simulink model "model"  (R2022a)
settings: Solver=VariableStepAuto  StartTime=0.0  StopTime=simtime  RelTol=1e-3
model workspace (MAT data in the model file):
  simtime = 3
values from neighbouring files (symbols this model uses):
  AVeh = 1.05    [first_test.mat]    (also in malgucka.m)
  coeffAir = 1.35    [first_test.mat]    (also in malgucka.m)
  coeffGrvy = 9.81    [first_test.mat]    (also in malgucka.m)
  coeffLift = 5.2    [first_test.mat]    (also in malgucka.m)
  coeffRoll = 0.025    [first_test.mat]    (also in malgucka.m)
  densAir = 1.225    [first_test.mat]    (also in malgucka.m)
  dstRdTir = 0.2032    [first_test.mat]    (also in malgucka.m)
  gbx = 16    [first_test.mat]    (also in malgucka.m = 13.11)
  initial_speed = max(v_acc) / 3.6    [laptimeV1.m]
  mTir = 5.3    [first_test.mat]    (also in malgucka.m)
  mVeh = 282    [first_test.mat]    (also in malgucka.m)
  tq_Mot_Re = [40 40 40 40 40 40 40 40 40 40 40 40 ... (46 elements, 1x46)]    [first_test.mat]    (also in laptimeV1.m = [0 0 0 0 0 0 0])
settings Model: Creator=gbour  LastModifiedBy=gbour
settings DebuggingCC: AlgebraicLoopMsg=none

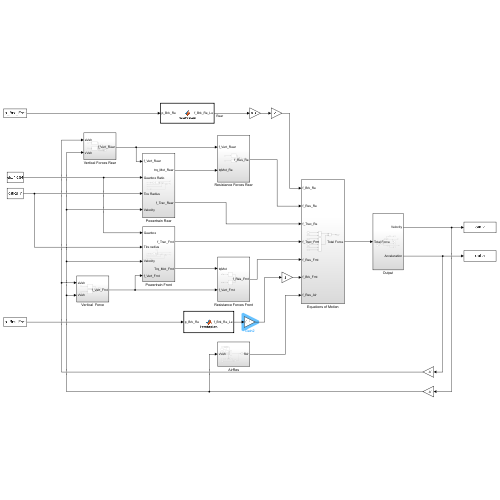
[thumbnail: Simulink's stored preview of the top-level diagram]
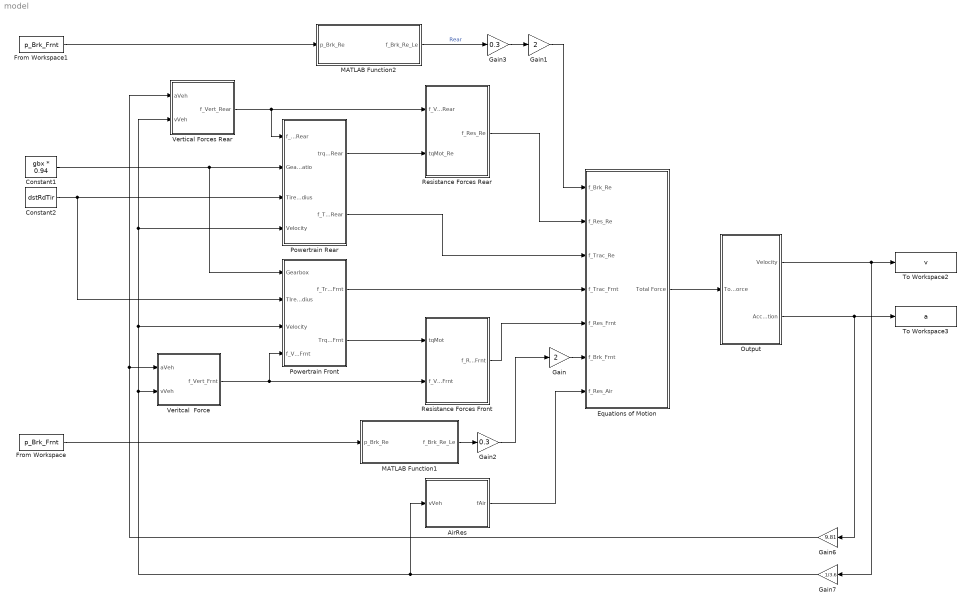
== system model ==
  AirRes : Subsystem
  Constant1 : Constant  Value=gbx * 0.94
  Constant2 : Constant  Value=dstRdTir
  Equations of Motion : Subsystem
  From Workspace : FromWorkspace  VariableName=p_Brk_Frnt
  From Workspace1 : FromWorkspace  VariableName=p_Brk_Frnt
  Gain : Gain  Gain=2
  Gain1 : Gain  Gain=2
  Gain2 : Gain  Gain=0.3
  Gain3 : Gain  Gain=0.3
  Gain6 : Gain  Gain=9.81
  Gain7 : Gain  Gain=1/3.6
  MATLAB Function1 : MATLAB Function  TreatAsAtomicUnit=on
  MATLAB Function2 : MATLAB Function  TreatAsAtomicUnit=on
  Output : Subsystem
  Powertrain Front : Subsystem
  Powertrain Rear : Subsystem
  Resistance Forces Front : Subsystem
  Resistance Forces Rear : Subsystem
  To Workspace2 : ToWorkspace  VariableName=v  SampleTime=-1
      settings: Save2DSignal=2-D array (concatenate along first dimension)
  To Workspace3 : ToWorkspace  VariableName=a  SampleTime=-1
      settings: Save2DSignal=2-D array (concatenate along first dimension)
  Veritcal  Force : Subsystem
  Vertical Forces Rear : Subsystem
  wires:
  Constant1/1 -> Powertrain Front/1(Gearbox), Powertrain Rear/2(Gearbox Ratio)
  Constant2/1 -> Powertrain Rear/3(Tire Radius), Powertrain Front/2(TIre radius)
  Output/1(Velocity) -> To Workspace2/1, Gain7/1
  Output/2(Acceleration) -> To Workspace3/1, Gain6/1
  Equations of Motion/1(Total Force) -> Output/1(Total Force)
  Resistance Forces Front/1(f_Res_Frnt) -> Equations of Motion/5(f_Res_Frnt)
  Veritcal  Force/1(f_Vert_Frnt) -> Powertrain Front/4(f_Vert_Frnt), Resistance Forces Front/2(f_Vert_Frnt)
  Powertrain Front/1(f_Trac_Frnt) -> Equations of Motion/4(f_Trac_Frnt)
  Powertrain Front/2(Trq_Mot_Frnt) -> Resistance Forces Front/1(tqMot)
  AirRes/1(fAir) -> Equations of Motion/7(f_Res_Air)
  Powertrain Rear/2(f_Trac_Rear) -> Equations of Motion/3(f_Trac_Re)
  Vertical Forces Rear/1(f_Vert_Rear) -> Resistance Forces Rear/1(f_Vert_Rear), Powertrain Rear/1(f_Vert_Rear)
  Powertrain Rear/1(trq_Mot_Rear) -> Resistance Forces Rear/2(tqMot_Re)
  Resistance Forces Rear/1(f_Res_Re) -> Equations of Motion/2(f_Res_Re)
  Gain6/1 -> Vertical Forces Rear/1(aVeh), Veritcal  Force/1(aVeh)
  Gain7/1 -> Powertrain Front/3(Velocity), Powertrain Rear/4(Velocity), Vertical Forces Rear/2(vVeh), Veritcal  Force/2(vVeh), AirRes/1(vVeh)
  MATLAB Function1/1(f_Brk_Re_Le) -> Gain2/1
  From Workspace/1 -> MATLAB Function1/1(p_Brk_Re)
  From Workspace1/1 -> MATLAB Function2/1(p_Brk_Re)
  MATLAB Function2/1(f_Brk_Re_Le) -> Gain3/1  "Rear"
  Gain/1 -> Equations of Motion/6(f_Brk_Frnt)
  Gain1/1 -> Equations of Motion/1(f_Brk_Re)
  Gain2/1 -> Gain/1
  Gain3/1 -> Gain1/1

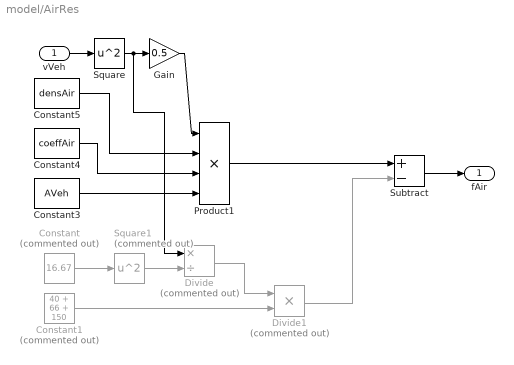
== system model/AirRes ==
  vVeh : Inport
  Constant : Constant  Commented=on  Value=16.67
  Constant1 : Constant  Commented=on  Value=40 + 66 + 150
  Constant3 : Constant  Value=AVeh
  Constant4 : Constant  Value=coeffAir
  Constant5 : Constant  Value=densAir
  Divide : Product  Commented=on  Inputs=*/
  Divide1 : Product  Commented=on  Inputs=**
  Gain : Gain  Gain=0.5
  Product1 : Product  Inputs=4
  Square : Math  Operator=square
  Square1 : Math  Commented=on  Operator=square
  Subtract : Sum  Inputs=+-
  fAir : Outport
  wires:
  Square/1 -> Divide/1, Gain/1
  Constant4/1 -> Product1/3
  Constant3/1 -> Product1/4
  Constant5/1 -> Product1/2
  vVeh/1 -> Square/1
  Gain/1 -> Product1/1
  Product1/1 -> Subtract/1
  Subtract/1 -> fAir/1
  Constant/1 -> Square1/1
  Square1/1 -> Divide/2
  Divide/1 -> Divide1/1
  Constant1/1 -> Divide1/2
  Divide1/1 -> Subtract/2

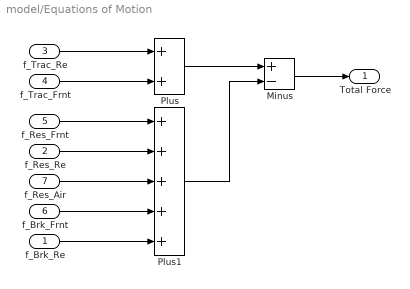
== system model/Equations of Motion ==
  f_Brk_Re : Inport
  f_Res_Re : Inport  Port=2
  f_Trac_Re : Inport  Port=3
  f_Trac_Frnt : Inport  Port=4
  f_Res_Frnt : Inport  Port=5
  f_Brk_Frnt : Inport  Port=6
  f_Res_Air : Inport  Port=7
  Minus : Sum  Inputs=+-
  Plus : Sum
  Plus1 : Sum  Inputs=+++++
  Total Force : Outport
  wires:
  f_Trac_Re/1 -> Plus/1
  f_Trac_Frnt/1 -> Plus/2
  f_Res_Frnt/1 -> Plus1/1
  f_Res_Re/1 -> Plus1/2
  Plus/1 -> Minus/1
  Plus1/1 -> Minus/2
  Minus/1 -> Total Force/1
  f_Res_Air/1 -> Plus1/3
  f_Brk_Frnt/1 -> Plus1/4
  f_Brk_Re/1 -> Plus1/5

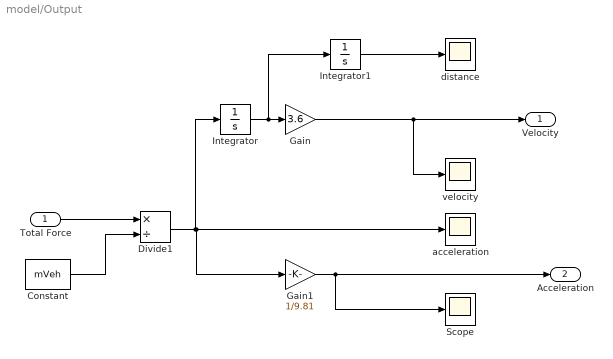
== system model/Output ==
  Total Force : Inport
  Constant : Constant  Value=mVeh
  Divide1 : Product  Inputs=*/
  Gain : Gain  Gain=3.6
  Gain1 : Gain  Gain=1/9.81
  Integrator : Integrator  InitialCondition=initial_speed
  Integrator1 : Integrator
  Scope : Scope
  acceleration : Scope
  distance : Scope
  velocity : Scope
  Velocity : Outport
  Acceleration : Outport  Port=2
  wires:
  Gain1/1 -> Acceleration/1, Scope/1
  Gain/1 -> Velocity/1, velocity/1
  Integrator1/1 -> distance/1
  Integrator/1 -> Gain/1, Integrator1/1
  Divide1/1 -> Integrator/1, acceleration/1, Gain1/1
  Constant/1 -> Divide1/2
  Total Force/1 -> Divide1/1

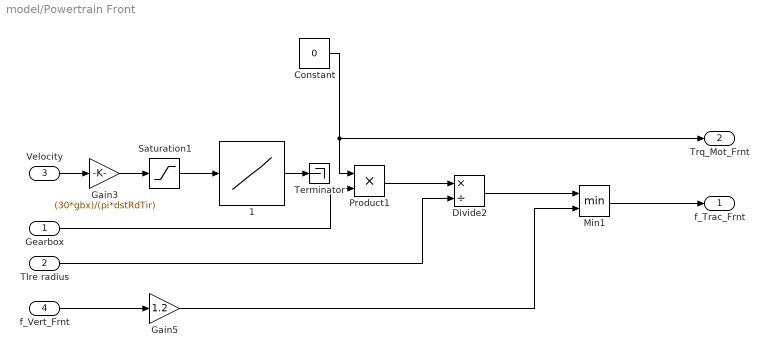
== system model/Powertrain Front ==
  Gearbox : Inport
  TIre radius : Inport  Port=2
  Velocity : Inport  Port=3
  f_Vert_Frnt : Inport  Port=4
  " 1" : Lookup_n-D  NumberOfTableDimensions=1  BreakpointsForDimension1=[0 100 12000 15000 20000 22500 22501]  Table=[29.1 29.1 29.1 26 18 15 0] .*2  InternalRulePriority=Speed  RndMeth=Simplest
  Constant : Constant  Value=0
  Divide2 : Product  Inputs=*/
  Gain3 : Gain  Gain=(30*gbx)/(pi*dstRdTir)
  Gain5 : Gain  Gain=1.2
  Min1 : MinMax  Inputs=2
  Product1 : Product
  Saturation1 : Saturate  UpperLimit=22501  LowerLimit=0
  Terminator : Terminator
  f_Trac_Frnt : Outport
  Trq_Mot_Frnt : Outport  Port=2
  wires:
  Gain5/1 -> Min1/2
  TIre radius/1 -> Divide2/2
  Gearbox/1 -> Product1/2
  Divide2/1 -> Min1/1
  Velocity/1 -> Gain3/1
  Product1/1 -> Divide2/1
  f_Vert_Frnt/1 -> Gain5/1
  Saturation1/1 -> " 1"/1
  Min1/1 -> f_Trac_Frnt/1
  Gain3/1 -> Saturation1/1
  " 1"/1 -> Terminator/1
  Constant/1 -> Trq_Mot_Frnt/1, Product1/1

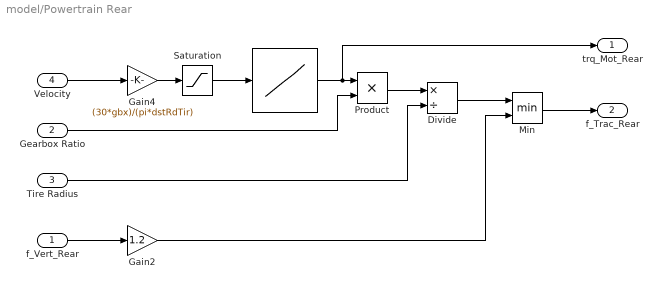
== system model/Powertrain Rear ==
  f_Vert_Rear : Inport
  Gearbox Ratio : Inport  Port=2
  Tire Radius : Inport  Port=3
  Velocity : Inport  Port=4
  " " : Lookup_n-D  NumberOfTableDimensions=1  BreakpointsForDimension1=[0 100 12000 15000 20000 22500 22501]  Table=tq_Mot_Re  InternalRulePriority=Speed  RndMeth=Simplest
  Divide : Product  Inputs=*/
  Gain2 : Gain  Gain=1.2
  Gain4 : Gain  Gain=(30*gbx)/(pi*dstRdTir)
  Min : MinMax  Inputs=2
  Product : Product
  Saturation : Saturate  UpperLimit=22501  LowerLimit=0
  trq_Mot_Rear : Outport
  f_Trac_Rear : Outport  Port=2
  wires:
  Product/1 -> Divide/1
  Tire Radius/1 -> Divide/2
  Gain2/1 -> Min/2
  Saturation/1 -> " "/1
  Gain4/1 -> Saturation/1
  " "/1 -> trq_Mot_Rear/1, Product/1
  Gearbox Ratio/1 -> Product/2
  Divide/1 -> Min/1
  Velocity/1 -> Gain4/1
  Min/1 -> f_Trac_Rear/1
  f_Vert_Rear/1 -> Gain2/1

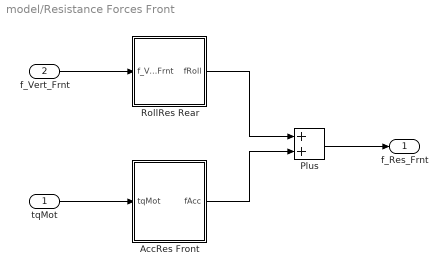
== system model/Resistance Forces Front ==
  tqMot : Inport
  f_Vert_Frnt : Inport  Port=2
  AccRes Front : Subsystem
  Plus : Sum
  RollRes Rear : Subsystem
  f_Res_Frnt : Outport
  wires:
  tqMot/1 -> AccRes Front/1(tqMot)
  Plus/1 -> f_Res_Frnt/1
  RollRes Rear/1(fRoll) -> Plus/1
  AccRes Front/1(fAcc) -> Plus/2
  f_Vert_Frnt/1 -> RollRes Rear/1(f_Vert_Frnt)

== system model/Resistance Forces Rear ==
  f_Vert_Rear : Inport
  tqMot_Re : Inport  Port=2
  AccRes : Subsystem
  Plus : Sum
  RollRes : Subsystem
  f_Res_Re : Outport
  wires:
  RollRes/1(fRoll) -> Plus/1
  AccRes/1(fAcc) -> Plus/2
  Plus/1 -> f_Res_Re/1
  f_Vert_Rear/1 -> RollRes/1(f_Vert_Rear)
  tqMot_Re/1 -> AccRes/1(tqMot)

== system model/Veritcal  Force ==
  aVeh : Inport
  vVeh : Inport  Port=2
  Plus : Sum
  Subsystem1 : Subsystem
  Weight Shift1 : Subsystem
  f_Vert_Frnt : Outport
  wires:
  Weight Shift1/1(fWeightShift) -> Plus/1
  aVeh/1 -> Weight Shift1/1(aVeh)
  vVeh/1 -> Subsystem1/1(vVeh)
  Plus/1 -> f_Vert_Frnt/1
  Subsystem1/1(fDwn) -> Plus/2

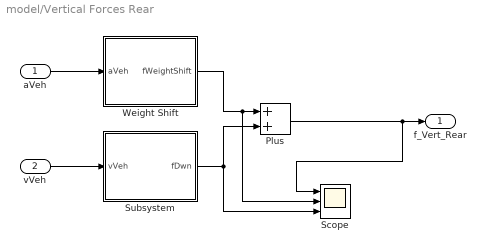
== system model/Vertical Forces Rear ==
  aVeh : Inport
  vVeh : Inport  Port=2
  Plus : Sum
  Scope : Scope  NumInputPorts=3
  Subsystem : Subsystem
  Weight Shift : Subsystem
  f_Vert_Rear : Outport
  wires:
  Weight Shift/1(fWeightShift) -> Scope/2, Plus/1
  Subsystem/1(fDwn) -> Plus/2, Scope/3
  aVeh/1 -> Weight Shift/1(aVeh)
  vVeh/1 -> Subsystem/1(vVeh)
  Plus/1 -> Scope/1, f_Vert_Rear/1

== system model/Resistance Forces Front/AccRes Front ==
  tqMot : Inport
  Constant : Constant  Value=dstRdTir
  Constant1 : Constant  Value=mTir
  Gain : Gain  Gain=1/4
  Product : Product  Inputs=3
  fAcc : Outport
  wires:
  tqMot/1 -> Gain/1
  Gain/1 -> Product/1
  Constant/1 -> Product/2
  Constant1/1 -> Product/3
  Product/1 -> fAcc/1

== system model/Resistance Forces Front/RollRes Rear ==
  f_Vert_Frnt : Inport
  Constant : Constant  Value=coeffRoll
  Gain : Gain  Gain=2
  Product : Product
  fRoll : Outport
  wires:
  Constant/1 -> Product/1
  Product/1 -> Gain/1
  f_Vert_Frnt/1 -> Product/2
  Gain/1 -> fRoll/1

== system model/Resistance Forces Rear/AccRes ==
  tqMot : Inport
  Constant : Constant  Value=dstRdTir
  Constant1 : Constant  Value=mTir
  Gain : Gain  Gain=1/4
  Product : Product  Inputs=3
  fAcc : Outport
  wires:
  tqMot/1 -> Gain/1
  Gain/1 -> Product/1
  Constant/1 -> Product/2
  Constant1/1 -> Product/3
  Product/1 -> fAcc/1

== system model/Resistance Forces Rear/RollRes ==
  f_Vert_Rear : Inport
  Constant : Constant  Value=coeffRoll
  Gain : Gain  Gain=2
  Product : Product
  fRoll : Outport
  wires:
  Constant/1 -> Product/1
  Product/1 -> Gain/1
  f_Vert_Rear/1 -> Product/2
  Gain/1 -> fRoll/1

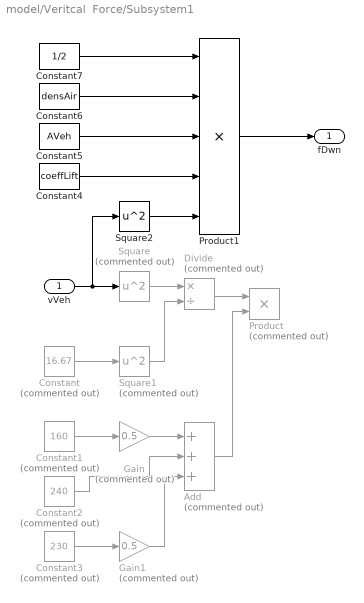
== system model/Veritcal  Force/Subsystem1 ==
  vVeh : Inport
  Add : Sum  Commented=on  Inputs=+++
  Constant : Constant  Commented=on  Value=16.67
  Constant1 : Constant  Commented=on  Value=160
  Constant2 : Constant  Commented=on  Value=240
  Constant3 : Constant  Commented=on  Value=230
  Constant4 : Constant  Value=coeffLift
  Constant5 : Constant  Value=AVeh
  Constant6 : Constant  Value=densAir
  Constant7 : Constant  Value=1/2
  Divide : Product  Commented=on  Inputs=*/
  Gain : Gain  Commented=on  Gain=0.5
  Gain1 : Gain  Commented=on  Gain=0.5
  Product : Product  Commented=on
  Product1 : Product  Inputs=5
  Square : Math  Commented=on  Operator=square
  Square1 : Math  Commented=on  Operator=square
  Square2 : Math  Operator=square
  fDwn : Outport
  wires:
  vVeh/1 -> Square2/1, Square/1
  Constant/1 -> Square1/1
  Square/1 -> Divide/1
  Square1/1 -> Divide/2
  Divide/1 -> Product/1
  Constant1/1 -> Gain/1
  Gain/1 -> Add/1
  Add/1 -> Product/2
  Constant3/1 -> Gain1/1
  Constant2/1 -> Add/2
  Gain1/1 -> Add/3
  Square2/1 -> Product1/5
  Constant4/1 -> Product1/4
  Constant5/1 -> Product1/3
  Constant6/1 -> Product1/2
  Constant7/1 -> Product1/1
  Product1/1 -> fDwn/1

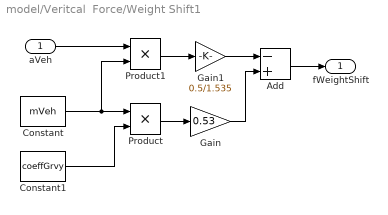
== system model/Veritcal  Force/Weight Shift1 ==
  aVeh : Inport
  Add : Sum  Inputs=-+
  Constant : Constant  Value=mVeh
  Constant1 : Constant  Value=coeffGrvy
  Gain : Gain  Gain=0.53
  Gain1 : Gain  Gain=0.5/1.535
  Product : Product
  Product1 : Product
  fWeightShift : Outport
  wires:
  Constant/1 -> Product1/2, Product/1
  Constant1/1 -> Product/2
  Product/1 -> Gain/1
  aVeh/1 -> Product1/1
  Product1/1 -> Gain1/1
  Gain1/1 -> Add/1
  Gain/1 -> Add/2
  Add/1 -> fWeightShift/1

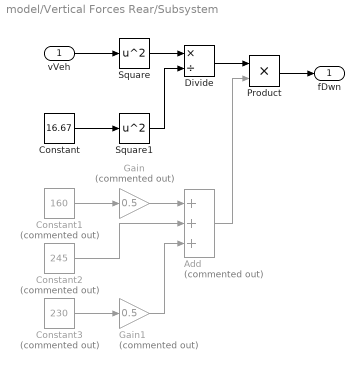
== system model/Vertical Forces Rear/Subsystem ==
  vVeh : Inport
  Add : Sum  Commented=on  Inputs=+++
  Constant : Constant  Value=16.67
  Constant1 : Constant  Commented=on  Value=160
  Constant2 : Constant  Commented=on  Value=245
  Constant3 : Constant  Commented=on  Value=230
  Divide : Product  Inputs=*/
  Gain : Gain  Commented=on  Gain=0.5
  Gain1 : Gain  Commented=on  Gain=0.5
  Product : Product
  Square : Math  Operator=square
  Square1 : Math  Operator=square
  fDwn : Outport
  wires:
  vVeh/1 -> Square/1
  Constant/1 -> Square1/1
  Square/1 -> Divide/1
  Square1/1 -> Divide/2
  Divide/1 -> Product/1
  Product/1 -> fDwn/1
  Constant1/1 -> Gain/1
  Gain/1 -> Add/1
  Add/1 -> Product/2
  Constant2/1 -> Add/2
  Constant3/1 -> Gain1/1
  Gain1/1 -> Add/3

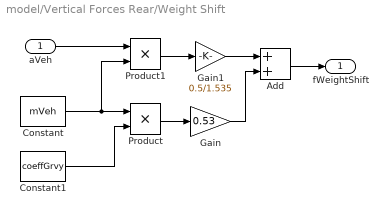
== system model/Vertical Forces Rear/Weight Shift ==
  aVeh : Inport
  Add : Sum
  Constant : Constant  Value=mVeh
  Constant1 : Constant  Value=coeffGrvy
  Gain : Gain  Gain=0.53
  Gain1 : Gain  Gain=0.5/1.535
  Product : Product
  Product1 : Product
  fWeightShift : Outport
  wires:
  Constant/1 -> Product1/2, Product/1
  Constant1/1 -> Product/2
  Product/1 -> Gain/1
  aVeh/1 -> Product1/1
  Product1/1 -> Gain1/1
  Gain1/1 -> Add/1
  Gain/1 -> Add/2
  Add/1 -> fWeightShift/1

== matlab function model/MATLAB Function2 ==
  data: p_Brk_Re input; f_Brk_Re_Le output
function f_Brk_Re_Le = rearbrakes(p_Brk_Re)

d_pi_r = 25.4;          % piston diameter rear [m]
nu_pi_r = 2;            % number of pistons rear
rad_brkdisc_r = 0.1725; % brakedisc radius rear [m]
mu_brk = 0.56;           % brake friction coefficient
rad_tir = 0.2032;          % tire radius [m]

f_Brk_Re_Le = (((pi * p_Brk_Re * ((d_pi_r^2)/4)) * nu_pi_r *mu_brk) * 0.5 * rad_brkdisc_r) / rad_tir;
end

== matlab function model/MATLAB Function1 ==
  data: p_Brk_Re input; f_Brk_Re_Le output
function f_Brk_Re_Le = frontbrakes(p_Brk_Re)

d_pi_r = 25.4;          % piston diameter rear [mm]
nu_pi_r = 4;            % number of pistons rear
rad_brkdisc_r = 0.1725; % brakedisc radius rear [m]
mu_brk = 0.56;          % brake friction coefficient
rad_tir = 0.2032;       % tire radius [m]

f_Brk_Re_Le = (((pi * p_Brk_Re * ((d_pi_r^2)/4)) * nu_pi_r *mu_brk) * 0.5 * rad_brkdisc_r) / rad_tir;
end
